simulink model "controller_testbench"  (R2022b)
settings: Solver=VariableStepAuto  StartTime=0.0  StopTime=10.0  RelTol=1e-3
model workspace (MAT data in the model file):
  Fz_stat_FL = Simulink.Parameter
  Fz_stat_FL.Value = 3921.3656
  Fz_stat_FL.DataType = 'double'
  Fz_stat_FL.DocUnits = 'N'
  Fz_stat_FL.Complexity = 'real'
  Fz_stat_FL.Dimensions = [1 1]
  Fz_stat_FR = Simulink.Parameter
  Fz_stat_FR.Value = 3921.3656
  Fz_stat_FR.DataType = 'double'
  Fz_stat_FR.DocUnits = 'N'
  Fz_stat_FR.Complexity = 'real'
  Fz_stat_FR.Dimensions = [1 1]
  Fz_stat_RL = Simulink.Parameter
  Fz_stat_RL.Value = 3922.1269
  Fz_stat_RL.DataType = 'double'
  Fz_stat_RL.DocUnits = 'N'
  Fz_stat_RL.Complexity = 'real'
  Fz_stat_RL.Dimensions = [1 1]
  Fz_stat_RR = Simulink.Parameter
  Fz_stat_RR.Value = 3922.1267
  Fz_stat_RR.DataType = 'double'
  Fz_stat_RR.DocUnits = 'N'
  Fz_stat_RR.Complexity = 'real'
  Fz_stat_RR.Dimensions = [1 1]
  cog_height = Simulink.Parameter
  cog_height.Value = 0.604
  cog_height.DataType = 'double'
  cog_height.DocUnits = 'm'
  cog_height.Complexity = 'real'
  cog_height.Dimensions = [1 1]
  g = Simulink.Parameter
  g.Value = 9.806
  g.DataType = 'double'
  g.DocUnits = 'm/s^2'
  g.Complexity = 'real'
  g.Dimensions = [1 1]
  lF = Simulink.Parameter
  lF.Value = 1.466
  lF.DataType = 'double'
  lF.DocUnits = 'm'
  lF.Complexity = 'real'
  lF.Dimensions = [1 1]
  lR = Simulink.Parameter
  lR.Value = 1.509
  lR.DataType = 'double'
  lR.DocUnits = 'm'
  lR.Complexity = 'real'
  lR.Dimensions = [1 1]
  pitchAngle = Simulink.Parameter
  pitchAngle.Value = [0.00443372596055 0.00472012698538 0.00500652801021 0.00529292903504 0.00557933005986 0.00586573108469 0.00615213210952 0.00643853313435 0.00672493415917 0.007011335184 0.00729773620883 0.00758413723366 ... (200 elements, 200x1)]
  pitchAngle.DataType = 'double'
  pitchAngle.DocUnits = 'rad'
  pitchAngle.Complexity = 'real'
  pitchAngle.Dimensions = [200 1]
  pitchStiffness = Simulink.Parameter
  pitchStiffness.Value = [286621.759635 286644.842257 286407.773968 286374.136656 286600.567598 286901.705993 287109.32323 287190.659823 287245.018359 287344.728913 287488.533524 287631.863692 ... (200 elements, 200x1)]
  pitchStiffness.DataType = 'double'
  pitchStiffness.DocUnits = 'N*m/rad'
  pitchStiffness.Complexity = 'real'
  pitchStiffness.Dimensions = [200 1]
  pitch_inertia = Simulink.Parameter
  pitch_inertia.Value = 2180.5
  pitch_inertia.DataType = 'double'
  pitch_inertia.DocUnits = 'kg * m^2'
  pitch_inertia.Complexity = 'real'
  pitch_inertia.Dimensions = [1 1]
  pitching_coefficient = Simulink.Parameter
  pitching_coefficient.Value = -0.002
  pitching_coefficient.DataType = 'double'
  pitching_coefficient.DocUnits = '1'
  pitching_coefficient.Complexity = 'real'
  pitching_coefficient.Dimensions = [1 1]
  rdyn = Simulink.Parameter
  rdyn.Value = 0.309
  rdyn.DataType = 'double'
  rdyn.DocUnits = 'm'
  rdyn.Complexity = 'real'
  rdyn.Dimensions = [1 1]
  reference_area = Simulink.Parameter
  reference_area.Value = 2.4
  reference_area.DataType = 'double'
  reference_area.DocUnits = 'kg / m^3'
  reference_area.Complexity = 'real'
  reference_area.Dimensions = [1 1]
  rho = Simulink.Parameter
  rho.Value = 1.2
  rho.DataType = 'double'
  rho.DocUnits = 'm^2'
  rho.Complexity = 'real'
  rho.Dimensions = [1 1]
  rollStiffness_F = Simulink.Parameter
  rollStiffness_F.Value = -66168.4036
  rollStiffness_F.DataType = 'double'
  rollStiffness_F.DocUnits = 'N*m/rad'
  rollStiffness_F.Complexity = 'real'
  rollStiffness_F.Dimensions = [1 1]
  rollStiffness_R = Simulink.Parameter
  rollStiffness_R.Value = -79058.3706
  rollStiffness_R.DataType = 'double'
  rollStiffness_R.DocUnits = 'N*m/rad'
  rollStiffness_R.Complexity = 'real'
  rollStiffness_R.Dimensions = [1 1]
  sprung_mass = Simulink.Parameter
  sprung_mass.Value = 1373.3
  sprung_mass.DataType = 'double'
  sprung_mass.DocUnits = 'kg'
  sprung_mass.Complexity = 'real'
  sprung_mass.Dimensions = [1 1]
  tire = Simulink.Parameter
  tire.Value.MDI_Header.FILE_VERSION = 2
  tire.Value.Model.USE_MODE = 14
  tire.Value.Dim.UNLOADED_RADIUS = 0.3185
  tire.Value.Dim.WIDTH = 0.205
  tire.Value.Dim.RIM_RADIUS = 0.1905
  tire.Value.Dim.RIM_WIDTH = 0.1524
  tire.Value.Dim.ASPECT_RATIO = 0.6
  tire.Value.Vertical.VERTICAL_STIFFNESS = 236700
  tire.Value.Vertical.VERTICAL_DAMPING = 50
  tire.Value.Vertical.BREFF = 5
  tire.Value.Vertical.DREFF = 0.3
  tire.Value.Vertical.FREFF = 0.1
  tire.Value.Vertical.FNOMIN = 6500
  tire.Value.Range.KPUMIN = -0.3
  tire.Value.Range.KPUMAX = 0.3
  tire.Value.Range.ALPMIN = -0.1745
  tire.Value.Range.ALPMAX = 0.1745
  tire.Value.Range.CAMMIN = -0.1047
  tire.Value.Range.CAMMAX = 0.1047
  tire.Value.Range.FZMIN = 400
  tire.Value.Range.FZMAX = 8500
  tire.Value.Scale.LFZO = 1
  tire.Value.Scale.LCX = 1
  tire.Value.Scale.LMUX = 1
  tire.Value.Scale.LEX = 1
  tire.Value.Scale.LKX = 1
  tire.Value.Scale.LHX = 1
  tire.Value.Scale.LVX = 1
  tire.Value.Scale.LGAX = 1
  tire.Value.Scale.LCY = 1
  tire.Value.Scale.LMUY = 1
  tire.Value.Scale.LEY = 1
  tire.Value.Scale.LKY = 1
  tire.Value.Scale.LHY = 1
  tire.Value.Scale.LVY = 1
  tire.Value.Scale.LGAY = 1
  tire.Value.Scale.LTR = 1
  tire.Value.Scale.LRES = 1
  tire.Value.Scale.LGAZ = 1
  tire.Value.Scale.LXAL = 1
  tire.Value.Scale.LYKA = 1
  tire.Value.Scale.LVYKA = 1
  tire.Value.Scale.LS = 1
  tire.Value.Scale.LSGKP = 1
  tire.Value.Scale.LSGAL = 1
  tire.Value.Scale.LGYR = 1
  tire.Value.Scale.LMX = 1
  tire.Value.Scale.LVMX = 1
  tire.Value.Scale.LMY = 1
  tire.Value.Long.PCX1 = 1.6055
  tire.Value.Long.PDX1 = 1.1703
  tire.Value.Long.PDX2 = -0.081328
  tire.Value.Long.PDX3 = 0
  tire.Value.Long.PEX1 = 0.53409
  tire.Value.Long.PEX2 = -0.019956
  tire.Value.Long.PEX3 = 0.18089
  tire.Value.Long.PEX4 = 2.9951e-07
  tire.Value.Long.PKX1 = 36.411
  tire.Value.Long.PKX2 = 0.12615
  tire.Value.Long.PKX3 = 0.51289
  tire.Value.Long.PHX1 = 0
  tire.Value.Long.PHX2 = 0
  tire.Value.Long.PVX1 = 0
  tire.Value.Long.PVX2 = 0
  tire.Value.Long.RBX1 = 18.456
  tire.Value.Long.RBX2 = 16.314
  tire.Value.Long.RCX1 = 1.091
  tire.Value.Long.REX1 = 0
  tire.Value.Long.REX2 = 0
  tire.Value.Long.RHX1 = 0.0058715
  tire.Value.Long.PTX1 = 1.5
  tire.Value.Long.PTX2 = 0.180096
  tire.Value.Long.PTX3 = -0.15
  tire.Value.OverTurn.QSX1 = 0.00023155
  tire.Value.OverTurn.QSX2 = 0.51574
  tire.Value.OverTurn.QSX3 = 0.046399
  tire.Value.Lat.PCY1 = 2.1322
  tire.Value.Lat.PDY1 = 1.0283
  tire.Value.Lat.PDY2 = -0.16758
  tire.Value.Lat.PDY3 = -1.5821
  tire.Value.Lat.PEY1 = 0.33443
  tire.Value.Lat.PEY2 = -1.8733
  tire.Value.Lat.PEY3 = -0.13136
  tire.Value.Lat.PEY4 = -11.677
  tire.Value.Lat.PKY1 = -20.505
  tire.Value.Lat.PKY2 = 2.0284
  tire.Value.Lat.PKY3 = 0.89994
  tire.Value.Lat.PHY1 = 0.0031377
  tire.Value.Lat.PHY2 = 0.00051596
  tire.Value.Lat.PHY3 = 0.039251
  tire.Value.Lat.PVY1 = 0.026365
  tire.Value.Lat.PVY2 = -0.0062119
  tire.Value.Lat.PVY3 = -0.41389
  tire.Value.Lat.PVY4 = -0.048038
  tire.Value.Lat.RBY1 = 22.003
  tire.Value.Lat.RBY2 = -13.623
  tire.Value.Lat.RBY3 = -0.0093616
  tire.Value.Lat.RCY1 = 0.98294
  tire.Value.Lat.REY1 = 0
  tire.Value.Lat.REY2 = 0
  tire.Value.Lat.RHY1 = -9.1492e-11
  tire.Value.Lat.RHY2 = 0
  tire.Value.Lat.RVY1 = 22.965
  tire.Value.Lat.RVY2 = 0.37981
  tire.Value.Lat.RVY3 = 1.8552
  tire.Value.Lat.RVY4 = 0.08767
  tire.Value.Lat.RVY5 = -8.8234e-11
  tire.Value.Lat.RVY6 = 0.90374
  tire.Value.Lat.PTY1 = 1.75
  tire.Value.Lat.PTY2 = 1.35
  tire.Value.Roll.QSY1 = 0.01
  tire.Value.Roll.QSY2 = 0
  tire.Value.Roll.QSY3 = 0
  tire.Value.Roll.QSY4 = 0
  tire.Value.Align.QBZ1 = 19.588
  tire.Value.Align.QBZ2 = -4.1671
  tire.Value.Align.QBZ3 = -0.34132
  tire.Value.Align.QBZ4 = -0.023607
  tire.Value.Align.QBZ5 = -0.0793
  tire.Value.Align.QBZ9 = -50
  tire.Value.Align.QBZ10 = 0
  tire.Value.Align.QCZ1 = 1.2012
  tire.Value.Align.QDZ1 = 0.12819
  tire.Value.Align.QDZ2 = -0.0052433
  tire.Value.Align.QDZ3 = -0.099544
  tire.Value.Align.QDZ4 = -15
  tire.Value.Align.QDZ6 = 6.2499e-05
  tire.Value.Align.QDZ7 = 0.00050135
  tire.Value.Align.QDZ8 = -0.28564
  tire.Value.Align.QDZ9 = -0.025056
  tire.Value.Align.QEZ1 = -0.0044308
  tire.Value.Align.QEZ2 = 0.022579
  tire.Value.Align.QEZ3 = -0.16199
  tire.Value.Align.QEZ4 = -0.5576
  tire.Value.Align.QEZ5 = -87.296
  tire.Value.Align.QHZ1 = 0.00082436
  tire.Value.Align.QHZ2 = 0.002733
  tire.Value.Align.QHZ3 = 0.15
  tire.Value.Align.QHZ4 = 0.11608
  tire.Value.Align.SSZ1 = -5.3899e-10
  tire.Value.Align.SSZ2 = -2.2371e-09
  tire.Value.Align.SSZ3 = 3.6029e-08
  tire.Value.Align.SSZ4 = 3.9826e-08
  tire.Value.Align.QTZ1 = 0.3
  tire.Value.Align.MBELT = 7.5
  tire.Value.FLoadMax = 10000
  tire.DataType = 'struct'
  tire.Complexity = 'real'
  tire.Dimensions = [1 1]
  total_pitchDamping = Simulink.Parameter
  total_pitchDamping.Value = 22000
  total_pitchDamping.DataType = 'double'
  total_pitchDamping.DocUnits = 'N*m/rad'
  total_pitchDamping.Complexity = 'real'
  total_pitchDamping.Dimensions = [1 1]
  total_pitchStiffness = Simulink.Parameter
  total_pitchStiffness.Value = 291158.1055
  total_pitchStiffness.DataType = 'double'
  total_pitchStiffness.DocUnits = 'N*m/rad'
  total_pitchStiffness.Complexity = 'real'
  total_pitchStiffness.Dimensions = [1 1]
  total_rollStiffness = Simulink.Parameter
  total_rollStiffness.Value = 138201.9734
  total_rollStiffness.DataType = 'double'
  total_rollStiffness.DocUnits = 'N*m/rad'
  total_rollStiffness.Complexity = 'real'
  total_rollStiffness.Dimensions = [1 1]
  trackwidth_F = Simulink.Parameter
  trackwidth_F.Value = 1.6
  trackwidth_F.DataType = 'double'
  trackwidth_F.DocUnits = 'm'
  trackwidth_F.Complexity = 'real'
  trackwidth_F.Dimensions = [1 1]
  trackwidth_R = Simulink.Parameter
  trackwidth_R.Value = 1.614
  trackwidth_R.DataType = 'double'
  trackwidth_R.DocUnits = 'm'
  trackwidth_R.Complexity = 'real'
  trackwidth_R.Dimensions = [1 1]
  unsprung_mass = Simulink.Parameter
  unsprung_mass.Value = 226.704
  unsprung_mass.DataType = 'double'
  unsprung_mass.DocUnits = 'kg'
  unsprung_mass.Complexity = 'real'
  unsprung_mass.Dimensions = [1 1]
  wheelbase = Simulink.Parameter
  wheelbase.Value = 2.975
  wheelbase.DataType = 'double'
  wheelbase.DocUnits = 'm'
  wheelbase.Complexity = 'real'
  wheelbase.Dimensions = [1 1]
settings Model: Creator=marcel  LastModifiedBy=marcel

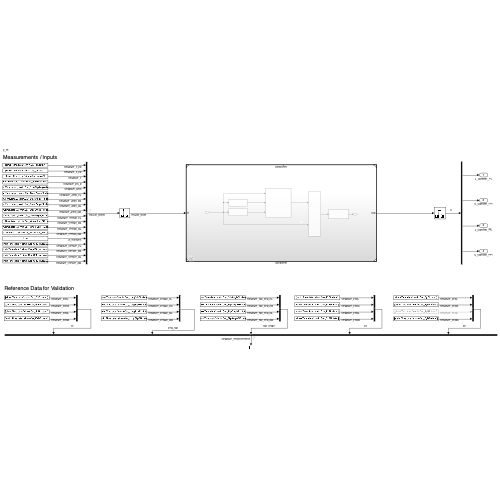
[thumbnail: Simulink's stored preview of the top-level diagram]
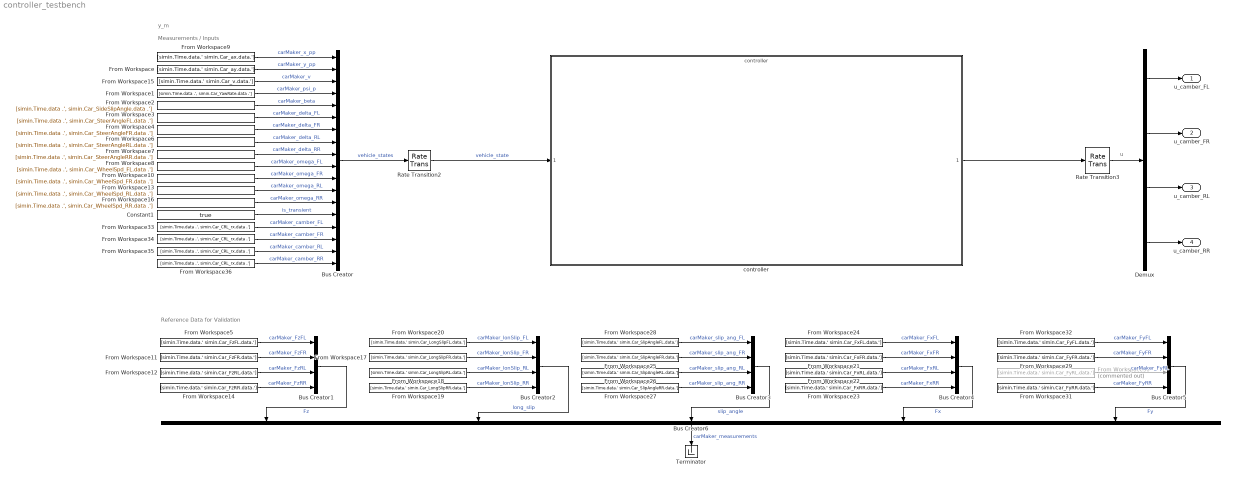
== system controller_testbench ==
  note: u
  note: y_m
  note: Reference Data for Validation
  note: Measurements / Inputs
  Bus Creator : BusCreator  Inputs=18  OutDataTypeStr=Bus: vehicle_states  NonVirtualBus=on
      settings: InheritFromInputs=off
  Bus Creator{1..5} (5 alike) : BusCreator  Inputs=4
  Bus Creator6 : BusCreator  Inputs=5
  Constant1 : Constant  Value=true  OutDataTypeStr=boolean  SampleTime=0.01
  Demux : Demux
  From Workspace : FromWorkspace  VariableName=[simin.Time.data.' simin.Car_ay.data.']  SampleTime=0.01
  From Workspace1 : FromWorkspace  VariableName=[simin.Time.data .', simin.Car_YawRate.data .']  SampleTime=0.01
  From Workspace10 : FromWorkspace  VariableName=[simin.Time.data .', simin.Car_WheelSpd_FR.data .']  SampleTime=0.01
  From Workspace11 : FromWorkspace  VariableName=[simin.Time.data.' simin.Car_FzFR.data.']  SampleTime=0.01
  From Workspace12 : FromWorkspace  VariableName=[simin.Time.data.' simin.Car_FzRL.data.']  SampleTime=0.01
  From Workspace13 : FromWorkspace  VariableName=[simin.Time.data .', simin.Car_WheelSpd_RL.data .']  SampleTime=0.01
  From Workspace14 : FromWorkspace  VariableName=[simin.Time.data.' simin.Car_FzRR.data.']  SampleTime=0.01
  From Workspace15 : FromWorkspace  VariableName=[simin.Time.data.' simin.Car_v.data.']  SampleTime=0.01
  From Workspace16 : FromWorkspace  VariableName=[simin.Time.data .', simin.Car_WheelSpd_RR.data .']  SampleTime=0.01
  From Workspace17 : FromWorkspace  VariableName=[simin.Time.data.' simin.Car_LongSlipFR.data.']  SampleTime=0.01
  From Workspace18 : FromWorkspace  VariableName=[simin.Time.data.' simin.Car_LongSlipRL.data.']  SampleTime=0.01
  From Workspace19 : FromWorkspace  VariableName=[simin.Time.data.' simin.Car_LongSlipRR.data.']  SampleTime=0.01
  From Workspace2 : FromWorkspace  VariableName=[simin.Time.data .', simin.Car_SideSlipAngle.data .']  SampleTime=0.01
  From Workspace20 : FromWorkspace  VariableName=[simin.Time.data.' simin.Car_LongSlipFL.data.']  SampleTime=0.01
  From Workspace21 : FromWorkspace  VariableName=[simin.Time.data.' simin.Car_FxFR.data.']  SampleTime=0.01
  From Workspace22 : FromWorkspace  VariableName=[simin.Time.data.' simin.Car_FxRL.data.']  SampleTime=0.01
  From Workspace23 : FromWorkspace  VariableName=[simin.Time.data.' simin.Car_FxRR.data.']  SampleTime=0.01
  From Workspace24 : FromWorkspace  VariableName=[simin.Time.data.' simin.Car_FxFL.data.']  SampleTime=0.01
  From Workspace25 : FromWorkspace  VariableName=[simin.Time.data.' simin.Car_SlipAngleFR.data.']  SampleTime=0.01
  From Workspace26 : FromWorkspace  VariableName=[simin.Time.data.' simin.Car_SlipAngleRL.data.']  SampleTime=0.01
  From Workspace27 : FromWorkspace  VariableName=[simin.Time.data.' simin.Car_SlipAngleRR.data.']  SampleTime=0.01
  From Workspace28 : FromWorkspace  VariableName=[simin.Time.data.' simin.Car_SlipAngleFL.data.']  SampleTime=0.01
  From Workspace29 : FromWorkspace  VariableName=[simin.Time.data.' simin.Car_FyFR.data.']  SampleTime=0.01
  From Workspace3 : FromWorkspace  VariableName=[simin.Time.data .', simin.Car_SteerAngleFL.data .']  SampleTime=0.01
  From Workspace30 : FromWorkspace  Commented=on  VariableName=[simin.Time.data.' simin.Car_FyRL.data.']  SampleTime=0.01
  From Workspace31 : FromWorkspace  VariableName=[simin.Time.data.' simin.Car_FyRR.data.']  SampleTime=0.01
  From Workspace32 : FromWorkspace  VariableName=[simin.Time.data.' simin.Car_FyFL.data.']  SampleTime=0.01
  From Workspace{33..36} (4 alike) : FromWorkspace  VariableName=[simin.Time.data .', simin.Car_CRL_rx.data .']  SampleTime=0.01
  From Workspace4 : FromWorkspace  VariableName=[simin.Time.data .', simin.Car_SteerAngleFR.data .']  SampleTime=0.01
  From Workspace5 : FromWorkspace  VariableName=[simin.Time.data.' simin.Car_FzFL.data.']  SampleTime=0.01
  From Workspace6 : FromWorkspace  VariableName=[simin.Time.data .', simin.Car_SteerAngleRL.data .']  SampleTime=0.01
  From Workspace7 : FromWorkspace  VariableName=[simin.Time.data .', simin.Car_SteerAngleRR.data .']  SampleTime=0.01
  From Workspace8 : FromWorkspace  VariableName=[simin.Time.data .', simin.Car_WheelSpd_FL.data .']  SampleTime=0.01
  From Workspace9 : FromWorkspace  VariableName=[simin.Time.data.' simin.Car_ax.data.']  SampleTime=0.01
  Rate Transition2 : RateTransition  OutPortSampleTime=0.001
  Rate Transition3 : RateTransition  OutPortSampleTime=0.001
  Terminator : Terminator
  controller : ModelReference  ModelNameDialog=controller.slx  SimulationMode=Normal  ModelReferenceVersion=1.3
  u_camber_FL : Outport
  u_camber_FR : Outport  Port=2
  u_camber_RL : Outport  Port=3
  u_camber_RR : Outport  Port=4
  wires:
  From Workspace9/1 -> Bus Creator/1  "carMaker_x_pp"
  From Workspace32/1 -> Bus Creator5/1  "carMaker_FyFL"
  From Workspace4/1 -> Bus Creator/7  "carMaker_delta_FR"
  From Workspace10/1 -> Bus Creator/11  "carMaker_omega_FR"
  Constant1/1 -> Bus Creator/14  "is_transient"
  From Workspace24/1 -> Bus Creator4/1  "carMaker_FxFL"
  Bus Creator4/1 -> Bus Creator6/4  "Fx"
  Demux/4 -> u_camber_RR/1
  From Workspace3/1 -> Bus Creator/6  "carMaker_delta_FL"
  From Workspace34/1 -> Bus Creator/16  "carMaker_camber_FR"
  From Workspace6/1 -> Bus Creator/8  "carMaker_delta_RL"
  From Workspace1/1 -> Bus Creator/4  "carMaker_psi_p"
  From Workspace25/1 -> Bus Creator3/2  "carMaker_slip_ang_FR"
  From Workspace2/1 -> Bus Creator/5  "carMaker_beta"
  Bus Creator2/1 -> Bus Creator6/2  "long_slip"
  From Workspace8/1 -> Bus Creator/10  "carMaker_omega_FL"
  Bus Creator3/1 -> Bus Creator6/3  "slip_angle"
  From Workspace23/1 -> Bus Creator4/4  "carMaker_FxRR"
  From Workspace11/1 -> Bus Creator1/2  "carMaker_FzFR"
  From Workspace21/1 -> Bus Creator4/2  "carMaker_FxFR"
  From Workspace5/1 -> Bus Creator1/1  "carMaker_FzFL"
  From Workspace31/1 -> Bus Creator5/4  "carMaker_FyRR"
  From Workspace30/1 -> Bus Creator5/3  "carMaker_FyRL"
  From Workspace35/1 -> Bus Creator/17  "carMaker_camber_RL"
  From Workspace20/1 -> Bus Creator2/1  "carMaker_lonSlip_FL"
  From Workspace28/1 -> Bus Creator3/1  "carMaker_slip_ang_FL"
  From Workspace/1 -> Bus Creator/2  "carMaker_y_pp"
  From Workspace14/1 -> Bus Creator1/4  "carMaker_FzRR"
  From Workspace36/1 -> Bus Creator/18  "carMaker_camber_RR"
  Bus Creator6/1 -> Terminator/1  "carMaker_measurements"
  From Workspace19/1 -> Bus Creator2/4  "carMaker_lonSlip_RR"
  From Workspace17/1 -> Bus Creator2/2  "carMaker_lonSlip_FR"
  From Workspace33/1 -> Bus Creator/15  "carMaker_camber_FL"
  From Workspace26/1 -> Bus Creator3/3  "carMaker_slip_ang_RL"
  From Workspace12/1 -> Bus Creator1/3  "carMaker_FzRL"
  Rate Transition3/1 -> Demux/1
  From Workspace18/1 -> Bus Creator2/3  "carMaker_lonSlip_RL"
  Bus Creator1/1 -> Bus Creator6/1  "Fz"
  From Workspace7/1 -> Bus Creator/9  "carMaker_delta_RR"
  From Workspace15/1 -> Bus Creator/3  "carMaker_v"
  Bus Creator/1 -> Rate Transition2/1  "vehicle_states"
  Demux/1 -> u_camber_FL/1
  From Workspace22/1 -> Bus Creator4/3  "carMaker_FxRL"
  Demux/3 -> u_camber_RL/1
  From Workspace27/1 -> Bus Creator3/4  "carMaker_slip_ang_RR"
  From Workspace13/1 -> Bus Creator/12  "carMaker_omega_RL"
  From Workspace29/1 -> Bus Creator5/2  "carMaker_FyFR"
  From Workspace16/1 -> Bus Creator/13  "carMaker_omega_RR"
  Demux/2 -> u_camber_FR/1
  Bus Creator5/1 -> Bus Creator6/5  "Fy"
  Rate Transition2/1 -> controller/1  "vehicle_state"
  controller/1 -> Rate Transition3/1
